simulink model "Controlled_speed"  (R2020b)
settings: Solver=VariableStepAuto  StartTime=0.0  StopTime=10.0  RelTol=1e-3
values from neighbouring files (symbols this model uses):
  b = 50.0    [PI_controller_data.sldd]
  ki = 30.0    [PI_controller_data.sldd]
  kp = 700.0    [PI_controller_data.sldd]
  M = 1000.0    [PI_controller_data.sldd]
settings Model: DataDictionary=PI_controller_data.sldd  Creator=DELL  LastModifiedBy=DELL
settings DataIOCC: SaveOutput=off  SaveTime=off

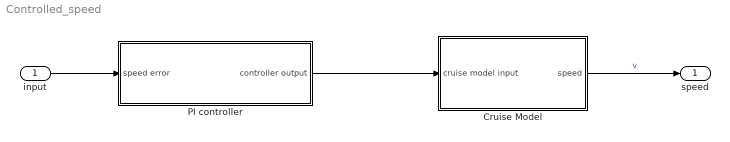
== system Controlled_speed ==
  input : Inport  OutDataTypeStr=double  PortDimensions=1  SampleTime=0
  Cruise Model : Subsystem
  PI controller : Subsystem
  speed : Outport  OutDataTypeStr=double  PortDimensions=1  SampleTime=0
  wires:
  PI controller/1(controller output) -> Cruise Model/1(cruise model input)
  input/1 -> PI controller/1(speed error)
  Cruise Model/1(speed) -> speed/1  "v"

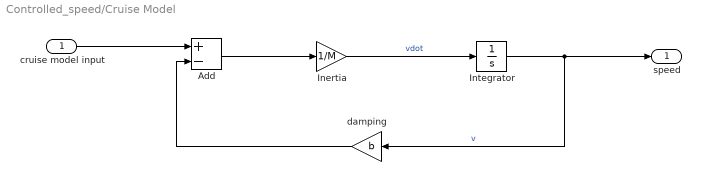
== system Controlled_speed/Cruise Model ==
  cruise model input : Inport
  Add : Sum  Inputs=+-
  Inertia : Gain  Gain=1/M
  Integrator : Integrator
  damping : Gain  Gain=b
  speed : Outport
  wires:
  Add/1 -> Inertia/1
  Inertia/1 -> Integrator/1  "vdot"
  cruise model input/1 -> Add/1
  damping/1 -> Add/2
  Integrator/1 -> damping/1, speed/1  "v"

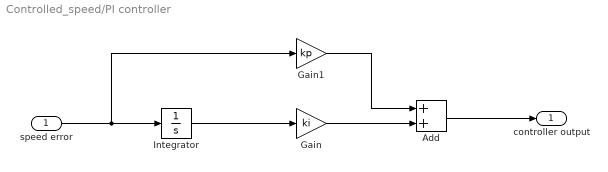
== system Controlled_speed/PI controller ==
  speed error : Inport
  Add : Sum
  Gain : Gain  Gain=ki
  Gain1 : Gain  Gain=kp
  Integrator : Integrator
  controller output : Outport
  wires:
  speed error/1 -> Integrator/1, Gain1/1
  Add/1 -> controller output/1
  Gain1/1 -> Add/1
  Integrator/1 -> Gain/1
  Gain/1 -> Add/2
